simulink model "Model"  (R2024b)
settings: Solver=ode45  StartTime=0.0  StopTime=10.0  RelTol=1e-3
InitFcn:
  | Main
values from neighbouring files (symbols this model uses):
  A = [0, 1; 0, -36]    [Main.m]
  B = [0; 180]    [Main.m]
  C = [1, 0]    [Main.m]
  D = 0    [Main.m]
  Go = [Gamma(2) - L*Gamma(1), Po * L + Phi(2, 1) - L * Phi(1, 1)]    [Main.m]
  Ho = [0; 1]    [Main.m]
  Jo = [0, 1; 0, L]    [Main.m]
  K = place(Phi, Gamma, Poles)    [Main.m]
  Nr = Nu + K * Nx    [Main.m]
  Po = Phi(2, 2) - L * Phi(1, 2)    [Main.m]
  Ts = 1e-3    (= 0.001)    [Main.m]
settings Model: Creator=Banaan  LastModifiedBy=Banaan

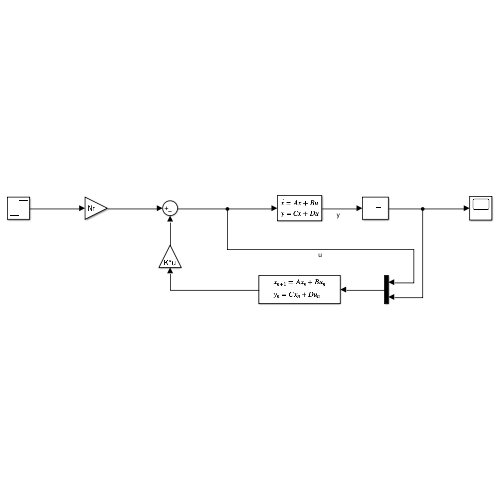
[thumbnail: Simulink's stored preview of the top-level diagram]
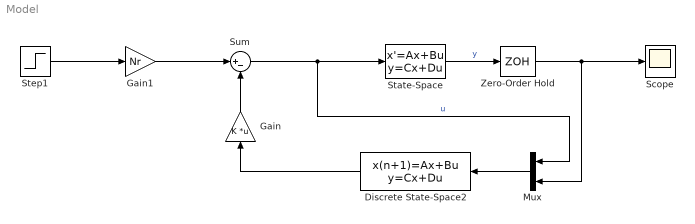
== system Model ==
  Discrete State-Space2 : DiscreteStateSpace  A=Po  B=Go  C=Ho  D=Jo  SampleTime=Ts
  Gain : Gain  Gain=K  Multiplication=Matrix(K*u)
  Gain1 : Gain  Gain=Nr
  Mux : Mux  Inputs=2
  Scope : Scope
  State-Space : StateSpace  A=A  B=B  C=C  D=D  InitialCondition=0
  Step1 : Step  SampleTime=0
  Sum : Sum  Inputs=|+-
  Zero-Order Hold : ZeroOrderHold  SampleTime=Ts
  wires:
  Mux/1 -> Discrete State-Space2/1
  Sum/1 -> State-Space/1, Mux/1  "u"
  State-Space/1 -> Zero-Order Hold/1  "y"
  Discrete State-Space2/1 -> Gain/1
  Gain/1 -> Sum/2
  Step1/1 -> Gain1/1
  Gain1/1 -> Sum/1
  Zero-Order Hold/1 -> Scope/1, Mux/2
